simulink model "rotors_pwm2"  (R2021a)
settings: Solver=FixedStepAuto  StartTime=0.0  StopTime=inf  RelTol=1e-3
libraries: robotlib x2
settings Model: Creator=chen  LastModifiedBy=chen
settings OptimizationCC: EnhancedBackFolding=on  PassReuseOutputArgsAs=Individual arguments  ZeroExternalMemoryAtStartup=off  ZeroInternalMemoryAtStartup=off  MaxStackSize=64  OptimizeBlockOrder=speed  DifferentSizesBufferReuse=on  OptimizationCustomize=off  EfficientTunableParamExpr=on
settings DebuggingCC: ParameterTunabilityLossMsg=error
settings HardwareCC: ProdBitPerPointer=32  ProdBitPerSizeT=32  ProdBitPerPtrDiffT=32  ProdLargestAtomicFloat=None  ProdIntDivRoundTo=Undefined  ProdEndianess=Unspecified  ProdWordSize=32  ProdHWDeviceType=Generic->Unspecified (assume 32-bit Generic)
settings SFSimCC: MATLABDynamicMemAlloc=off
settings RTWCC: SystemTargetFile=ert.tlc  HardwareBoard=Robot Operating System (ROS)  TLCOptions="-aInlineSetEventsForThisBaseRateFcn=TLC_FALSE -aSuppressMultiTaskScheduler=TLC_FALSE  -aRateBasedStepFcn=0"  TemplateMakefile=ert_default_tmf  Toolchain=Catkin  TargetLang=C++
settings CodeAppCC: ForceParamTrailComments=on  IgnoreCustomStorageClasses=off  OperatorAnnotations=on  SimulinkDataObjDesc=on  SFDataObjDesc=on  InsertBlockDesc=on

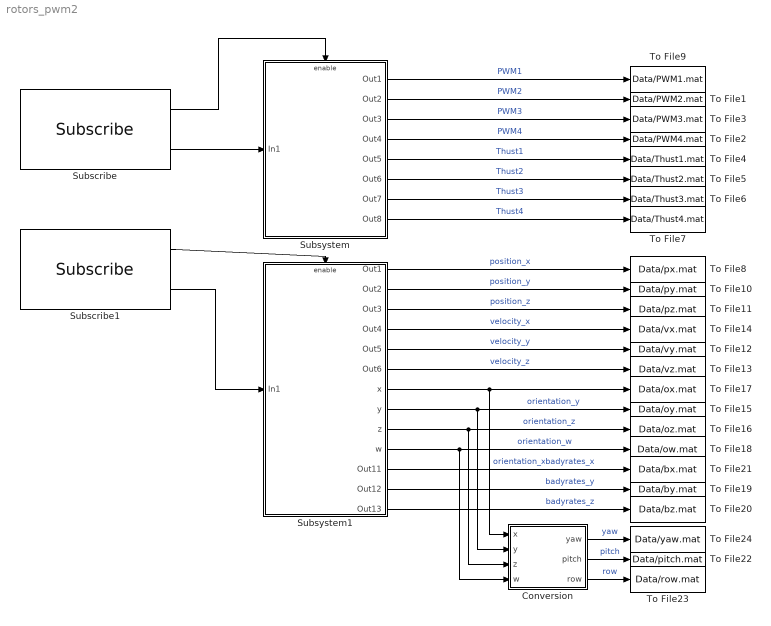
== system rotors_pwm2 ==
  Conversion : MATLAB Function  TreatAsAtomicUnit=on
  Subscribe : robotlib/Subscribe  topicSource=Select from ROS network  topic=/hummingbird/control_command  messageType=quad_msgs/ControlCommand  SampleTime=-1  legacyBusStruct=off  messageQueueLength=1
  Subscribe1 : robotlib/Subscribe  topicSource=Select from ROS network  topic=/hummingbird/state_est  messageType=quad_msgs/QuadStateEstimate  SampleTime=-1  legacyBusStruct=off  messageQueueLength=1
  Subsystem : Subsystem
  Subsystem1 : Subsystem
  To File1 : ToFile  Filename=Data/PWM2.mat  MatrixName=PWM2
  To File10 : ToFile  Filename=Data/py.mat  MatrixName=py
  To File11 : ToFile  Filename=Data/pz.mat  MatrixName=pz
  To File12 : ToFile  Filename=Data/vy.mat  MatrixName=vy
  To File13 : ToFile  Filename=Data/vz.mat  MatrixName=vz
  To File14 : ToFile  Filename=Data/vx.mat  MatrixName=vx
  To File15 : ToFile  Filename=Data/oy.mat  MatrixName=oy
  To File16 : ToFile  Filename=Data/oz.mat  MatrixName=oz
  To File17 : ToFile  Filename=Data/ox.mat  MatrixName=ox
  To File18 : ToFile  Filename=Data/ow.mat  MatrixName=ow
  To File19 : ToFile  Filename=Data/by.mat  MatrixName=by
  To File2 : ToFile  Filename=Data/PWM4.mat  MatrixName=PWM4
  To File20 : ToFile  Filename=Data/bz.mat  MatrixName=bz
  To File21 : ToFile  Filename=Data/bx.mat  MatrixName=bx
  To File22 : ToFile  Filename=Data/pitch.mat  MatrixName=pitch
  To File23 : ToFile  Filename=Data/row.mat  MatrixName=row
  To File24 : ToFile  Filename=Data/yaw.mat  MatrixName=yaw
  To File3 : ToFile  Filename=Data/PWM3.mat  MatrixName=PWM3
  To File4 : ToFile  Filename=Data/Thust1.mat  MatrixName=Thust1
  To File5 : ToFile  Filename=Data/Thust2.mat  MatrixName=Thust2
  To File6 : ToFile  Filename=Data/Thust3.mat  MatrixName=Thust3
  To File7 : ToFile  Filename=Data/Thust4.mat  MatrixName=Thust4
  To File8 : ToFile  Filename=Data/px.mat  MatrixName=px
  To File9 : ToFile  Filename=Data/PWM1.mat  MatrixName=PWM1
  wires:
  Subscribe/2 -> Subsystem/1(In1)
  Subscribe/1 -> Subsystem/Enable
  Subsystem/1(Out1) -> To File9/1  "PWM1"
  Subsystem/2(Out2) -> To File1/1  "PWM2"
  Subsystem/3(Out3) -> To File3/1  "PWM3"
  Subsystem/4(Out4) -> To File2/1  "PWM4"
  Subsystem/5(Out5) -> To File4/1  "Thust1"
  Subsystem/6(Out6) -> To File5/1  "Thust2"
  Subsystem/7(Out7) -> To File6/1  "Thust3"
  Subsystem/8(Out8) -> To File7/1  "Thust4"
  Subscribe1/2 -> Subsystem1/1(In1)
  Subscribe1/1 -> Subsystem1/Enable
  Subsystem1/1(Out1) -> To File8/1  "position_x"
  Subsystem1/2(Out2) -> To File10/1  "position_y"
  Subsystem1/3(Out3) -> To File11/1  "position_z"
  Subsystem1/6(Out6) -> To File13/1  "velocity_z"
  Subsystem1/5(Out5) -> To File12/1  "velocity_y"
  Subsystem1/4(Out4) -> To File14/1  "velocity_x"
  Subsystem1/7(x) -> To File17/1, Conversion/1(x)  "orientation_x"
  Subsystem1/8(y) -> To File15/1, Conversion/2(y)  "orientation_y"
  Subsystem1/9(z) -> To File16/1, Conversion/3(z)  "orientation_z"
  Subsystem1/10(w) -> To File18/1, Conversion/4(w)  "orientation_w"
  Subsystem1/11(Out11) -> To File21/1  "badyrates_x"
  Subsystem1/12(Out12) -> To File19/1  "badyrates_y"
  Subsystem1/13(Out13) -> To File20/1  "badyrates_z"
  Conversion/1(yaw) -> To File24/1  "yaw"
  Conversion/2(pitch) -> To File22/1  "pitch"
  Conversion/3(row) -> To File23/1  "row"

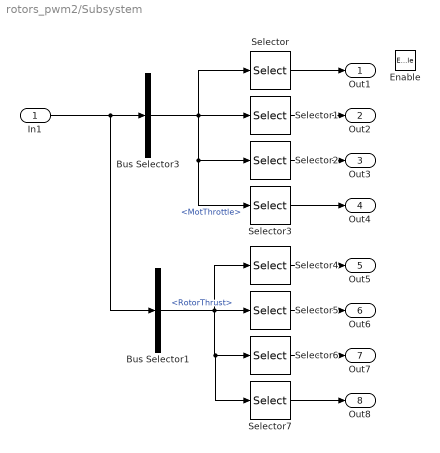
== system rotors_pwm2/Subsystem ==
  In1 : Inport
  Enable : EnablePort
  Bus Selector1 : BusSelector  OutputSignals=RotorThrust
  Bus Selector3 : BusSelector  OutputSignals=MotThrottle
  Selector : Selector  NumberOfDimensions=2  InputPortWidth=3  IndexOptions=Index vector (dialog),Index vector (dialog)  Indices=1,1  OutputSizes=1,1
  Selector1 : Selector  NumberOfDimensions=2  InputPortWidth=3  IndexOptions=Index vector (dialog),Index vector (dialog)  Indices=2,1  OutputSizes=1,1
  Selector2 : Selector  NumberOfDimensions=2  InputPortWidth=3  IndexOptions=Index vector (dialog),Index vector (dialog)  Indices=3,1  OutputSizes=1,1
  Selector3 : Selector  NumberOfDimensions=2  InputPortWidth=3  IndexOptions=Index vector (dialog),Index vector (dialog)  Indices=4,1  OutputSizes=1,1
  Selector4 : Selector  NumberOfDimensions=2  InputPortWidth=3  IndexOptions=Index vector (dialog),Index vector (dialog)  Indices=1,1  OutputSizes=1,1
  Selector5 : Selector  NumberOfDimensions=2  InputPortWidth=3  IndexOptions=Index vector (dialog),Index vector (dialog)  Indices=2,1  OutputSizes=1,1
  Selector6 : Selector  NumberOfDimensions=2  InputPortWidth=3  IndexOptions=Index vector (dialog),Index vector (dialog)  Indices=3,1  OutputSizes=1,1
  Selector7 : Selector  NumberOfDimensions=2  InputPortWidth=3  IndexOptions=Index vector (dialog),Index vector (dialog)  Indices=4,1  OutputSizes=1,1
  Out1 : Outport
  Out2 : Outport  Port=2
  Out3 : Outport  Port=3
  Out4 : Outport  Port=4
  Out5 : Outport  Port=5
  Out6 : Outport  Port=6
  Out7 : Outport  Port=7
  Out8 : Outport  Port=8
  wires:
  Selector/1 -> Out1/1
  Selector1/1 -> Out2/1
  Selector2/1 -> Out3/1
  Selector3/1 -> Out4/1
  In1/1 -> Bus Selector1/1, Bus Selector3/1
  Bus Selector3/1 -> Selector3/1, Selector2/1, Selector/1, Selector1/1  "<MotThrottle>"
  Selector7/1 -> Out8/1
  Selector6/1 -> Out7/1
  Selector5/1 -> Out6/1
  Selector4/1 -> Out5/1
  Bus Selector1/1 -> Selector7/1, Selector6/1, Selector4/1, Selector5/1  "<RotorThrust>"

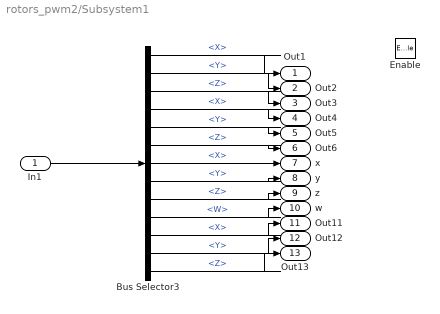
== system rotors_pwm2/Subsystem1 ==
  In1 : Inport
  Enable : EnablePort
  Bus Selector3 : BusSelector  OutputSignals=Position.X,Position.Y,Position.Z,Velocity.X,Velocity.Y,Velocity.Z,Orientation.X,Orientation.Y,Orientation.Z,Orientation.W,Bodyrates.X,Bodyrates.Y,Bodyrates.Z
  Out1 : Outport
  Out2 : Outport  Port=2
  Out3 : Outport  Port=3
  Out4 : Outport  Port=4
  Out5 : Outport  Port=5
  Out6 : Outport  Port=6
  x : Outport  Port=7
  y : Outport  Port=8
  z : Outport  Port=9
  w : Outport  Port=10
  Out11 : Outport  Port=11
  Out12 : Outport  Port=12
  Out13 : Outport  Port=13
  wires:
  In1/1 -> Bus Selector3/1
  Bus Selector3/3 -> Out3/1  "<Z>"
  Bus Selector3/2 -> Out2/1  "<Y>"
  Bus Selector3/1 -> Out1/1  "<X>"
  Bus Selector3/4 -> Out4/1  "<X>"
  Bus Selector3/5 -> Out5/1  "<Y>"
  Bus Selector3/6 -> Out6/1  "<Z>"
  Bus Selector3/7 -> x/1  "<X>"
  Bus Selector3/8 -> y/1  "<Y>"
  Bus Selector3/9 -> z/1  "<Z>"
  Bus Selector3/10 -> w/1  "<W>"
  Bus Selector3/11 -> Out11/1  "<X>"
  Bus Selector3/12 -> Out12/1  "<Y>"
  Bus Selector3/13 -> Out13/1  "<Z>"

== matlab function rotors_pwm2/Conversion ==
  data: yaw output; x input; y input; z input; w input; pitch output; row output
function [yaw,pitch,row] = quat2eul(x,y,z,w)
%#codegen

% Convert the quaternion to a yaw angle (zyx euler angle)
eul = quat2eul([w,x,y,z]);
yaw = eul(1);
pitch = eul(2);
row = eul(3);
end
